simulink model "QArm_PickPlace_v2"  (R2024b)
settings: Solver=ode45  StartTime=0.0  StopTime=11  MaxStep=0.05  RelTol=1e-4  AbsTol=1e-6
settings Model: Creator=Zohaib Ahmed Mughal  LastModifiedBy=Zohaib Ahmed Mughal

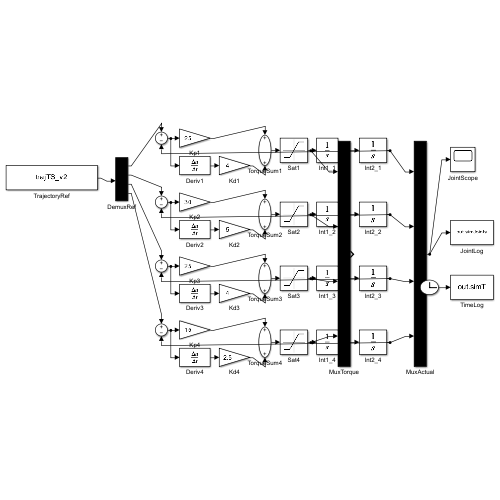
[thumbnail: Simulink's stored preview of the top-level diagram]
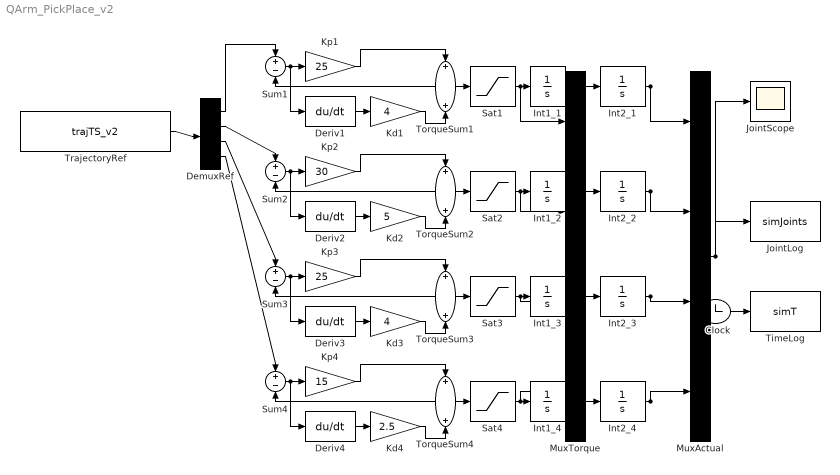
== system QArm_PickPlace_v2 ==
  Clock : Clock
  DemuxRef : Demux
  Deriv{1..4} (4 alike) : Derivative
  Int1_{1..4} (4 alike) : Integrator
  Int2_{1..4} (4 alike) : Integrator
  JointLog : ToWorkspace  VariableName=simJoints  SampleTime=-1
  JointScope : Scope
  Kd1 : Gain  Gain=4
  Kd2 : Gain  Gain=5
  Kd3 : Gain  Gain=4
  Kd4 : Gain  Gain=2.5
  Kp1 : Gain  Gain=25
  Kp2 : Gain  Gain=30
  Kp3 : Gain  Gain=25
  Kp4 : Gain  Gain=15
  MuxActual : Mux
  MuxTorque : Mux
  Sat{1..4} (4 alike) : Saturate  UpperLimit=15  LowerLimit=-15
  Sum{1..4} (4 alike) : Sum  Inputs=+-
  TimeLog : ToWorkspace  VariableName=simT  SampleTime=-1
  TorqueSum{1..4} (4 alike) : Sum
  TrajectoryRef : FromWorkspace  VariableName=trajTS_v2
  wires:
  TrajectoryRef/1 -> DemuxRef/1
  DemuxRef/1 -> Sum1/1
  Sum1/1 -> Kp1/1, Deriv1/1
  Kp1/1 -> TorqueSum1/1
  Deriv1/1 -> Kd1/1
  Kd1/1 -> TorqueSum1/2
  TorqueSum1/1 -> Sat1/1
  Sat1/1 -> Int1_1/1, MuxTorque/1
  Int1_1/1 -> Int2_1/1
  Int2_1/1 -> Sum1/2, MuxActual/1
  DemuxRef/2 -> Sum2/1
  Sum2/1 -> Kp2/1, Deriv2/1
  Kp2/1 -> TorqueSum2/1
  Deriv2/1 -> Kd2/1
  Kd2/1 -> TorqueSum2/2
  TorqueSum2/1 -> Sat2/1
  Sat2/1 -> Int1_2/1, MuxTorque/2
  Int1_2/1 -> Int2_2/1
  Int2_2/1 -> Sum2/2, MuxActual/2
  DemuxRef/3 -> Sum3/1
  Sum3/1 -> Kp3/1, Deriv3/1
  Kp3/1 -> TorqueSum3/1
  Deriv3/1 -> Kd3/1
  Kd3/1 -> TorqueSum3/2
  TorqueSum3/1 -> Sat3/1
  Sat3/1 -> Int1_3/1, MuxTorque/3
  Int1_3/1 -> Int2_3/1
  Int2_3/1 -> Sum3/2, MuxActual/3
  DemuxRef/4 -> Sum4/1
  Sum4/1 -> Kp4/1, Deriv4/1
  Kp4/1 -> TorqueSum4/1
  Deriv4/1 -> Kd4/1
  Kd4/1 -> TorqueSum4/2
  TorqueSum4/1 -> Sat4/1
  Sat4/1 -> Int1_4/1, MuxTorque/4
  Int1_4/1 -> Int2_4/1
  Int2_4/1 -> Sum4/2, MuxActual/4
  MuxActual/1 -> JointScope/1, JointLog/1
  Clock/1 -> TimeLog/1
